simulink model "model1"  (R2021b)
settings: Solver=VariableStepAuto  StartTime=0.0  StopTime=10.0  RelTol=1e-3
undefined symbols (not defined in the file): A, B, C, D
settings Model: Creator=szczy  LastModifiedBy=szczy

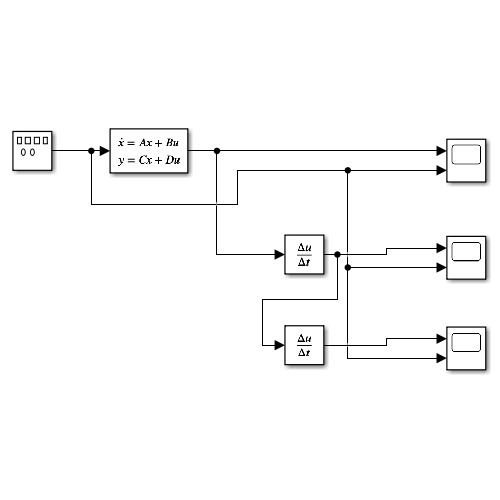
[thumbnail: Simulink's stored preview of the top-level diagram]
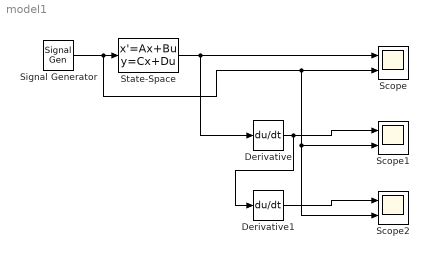
== system model1 ==
  Derivative : Derivative
  Derivative1 : Derivative
  Scope : Scope  NumInputPorts=2
  Scope1 : Scope  NumInputPorts=2
  Scope2 : Scope  NumInputPorts=2
  Signal Generator : SignalGenerator  WaveForm=square  Units=rad/sec
  State-Space : StateSpace  A=A  B=B  C=C  D=D  InitialCondition=0
  wires:
  Signal Generator/1 -> Scope2/2, Scope1/2, Scope/2, State-Space/1
  State-Space/1 -> Derivative/1, Scope/1
  Derivative/1 -> Derivative1/1, Scope1/1
  Derivative1/1 -> Scope2/1
